simulink model "CORDIC_SAP"  (R2021a)
settings: Solver=VariableStepAuto  StartTime=0.0  StopTime=10.0  RelTol=1e-3
undefined symbols (not defined in the file or in its folder): AXI4, Lite
libraries: hdlBasic x278, xbsIndex_r4 x1
(part 3 of 3)

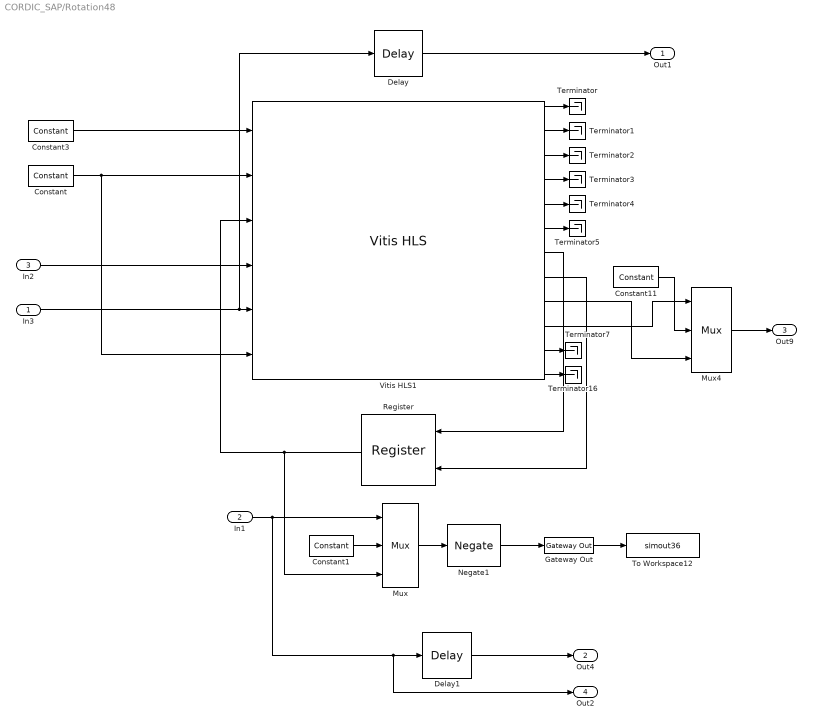
== system CORDIC_SAP/Rotation48 ==
  In3 : Inport
  In1 : Inport  Port=2
  In2 : Inport  Port=3
  Constant : hdlBasic/Constant  const=1.0  gui_display_data_type=Boolean  arith_type=Boolean  n_bits=16  bin_pt=14  preci_type=Single  exp_width=8  frac_width=24  explicit_period=off  period=1  XmcBlockStatus=1  maskContainerNames=tabcontainer1  block_type=constant  block_config=sysgen:Constant_config
  Constant1 : hdlBasic/Constant  const=0  gui_display_data_type=Fixed-point  arith_type=Signed (2's comp)  n_bits=16  bin_pt=13  preci_type=Single  exp_width=8  frac_width=24  explicit_period=off  period=1  XmcBlockStatus=1  maskContainerNames=tabcontainer1  block_type=constant  block_config=sysgen:Constant_config
  Constant11 : hdlBasic/Constant  const=0  gui_display_data_type=Fixed-point  arith_type=Signed (2's comp)  n_bits=16  bin_pt=13  preci_type=Single  exp_width=8  frac_width=24  explicit_period=off  period=1  XmcBlockStatus=1  maskContainerNames=tabcontainer1  block_type=constant  block_config=sysgen:Constant_config
  Constant3 : hdlBasic/Constant  const=0  gui_display_data_type=Boolean  arith_type=Boolean  n_bits=16  bin_pt=14  preci_type=Single  exp_width=8  frac_width=24  explicit_period=off  period=1  XmcBlockStatus=1  maskContainerNames=tabcontainer1  block_type=constant  block_config=sysgen:Constant_config
  Delay : hdlBasic/Delay  rst=off  en=off  latency=27  reg_retiming=off  XmcBlockStatus=1  maskContainerNames=group1  block_type=delay  block_config=sysgen:Delay_config
  Delay1 : hdlBasic/Delay  rst=off  en=off  latency=27  reg_retiming=off  XmcBlockStatus=1  maskContainerNames=group1  block_type=delay  block_config=sysgen:Delay_config
  Gateway Out : hdlBasic/Gateway Out  inherit_from_input=off  hdl_port=on  rows=1  columns=1  UseAsDAC=off  DACChannel='1'  interface=AXI4-Lite  automatic_assignment=on  address_offset=hex2dec('00')  intf_name=''  intf_description='Q_3_1'  timing_constraint=None  locs_specified=off  LOCs={}  io_standard={}  XmcBlockStatus=1  maskContainerNames=group4  block_type=gatewayout  block_config=sysgen:gateway_out_config  block_width_w=590  block_height_w=620  block_width=620  block_height=750
  Mux : hdlBasic/Mux  inputs=2  en=off  latency=1  precision=Full  arith_type=Unsigned  n_bits=16  bin_pt=14  quantization=Truncate  overflow=Wrap  XmcBlockStatus=1  maskContainerNames=tabcontainer1  block_type=mux  block_config=sysgen:Mux_config
  Mux4 : hdlBasic/Mux  inputs=2  en=off  latency=1  precision=Full  arith_type=Unsigned  n_bits=16  bin_pt=14  quantization=Truncate  overflow=Wrap  XmcBlockStatus=1  maskContainerNames=tabcontainer1  block_type=mux  block_config=sysgen:Mux_config
  Negate1 : hdlBasic/Negate  precision=Full  arith_type=Unsigned  n_bits=16  bin_pt=14  quantization=Truncate  overflow=Wrap  en=off  latency=0  XmcBlockStatus=1  maskContainerNames=tabcontainer1  block_type=negate  block_config=sysgen:Negate_config
  Register : hdlBasic/Register  init=0  rst=off  en=on  XmcBlockStatus=1  maskContainerNames=tabcontainer1  block_type=register  block_config=sysgen:Register_config
  Terminator{,1..5,7,16} (8 alike) : Terminator
  To Workspace12 : ToWorkspace  VariableName=simout36  SaveFormat=Timeseries  SampleTime=-1
  Vitis HLS1 : hdlBasic/Vitis HLS  anytable='C:\ELEC522\jz118\HLS\cordic\solution1'  fast_sim=off  display_datatype=off  rate_propagation_method=Simulink system period  model_file_path=''  latency=1  block_type=vitis_hls
      settings: infoedit=This block allows including C,C++ and SystemC source files in System Generator for DSP designs.
  Out1 : Outport
  Out4 : Outport  Port=2
  Out9 : Outport  Port=3
  Out2 : Outport  Port=4
  wires:
  In2/1 -> Vitis HLS1/4
  In3/1 -> Delay/1, Vitis HLS1/5
  Delay/1 -> Out1/1
  Constant/1 -> Vitis HLS1/2, Vitis HLS1/6
  Constant3/1 -> Vitis HLS1/1
  Vitis HLS1/1 -> Terminator/1
  Vitis HLS1/2 -> Terminator1/1
  Vitis HLS1/3 -> Terminator2/1
  Vitis HLS1/4 -> Terminator3/1
  Vitis HLS1/5 -> Terminator4/1
  Vitis HLS1/6 -> Terminator5/1
  Vitis HLS1/11 -> Terminator7/1
  Vitis HLS1/12 -> Terminator16/1
  Register/1 -> Mux/3, Vitis HLS1/3
  Vitis HLS1/8 -> Register/2
  Vitis HLS1/7 -> Register/1
  Constant11/1 -> Mux4/2
  Mux4/1 -> Out9/1
  Vitis HLS1/9 -> Mux4/3
  Vitis HLS1/10 -> Mux4/1
  In1/1 -> Out2/1, Delay1/1, Mux/1
  Constant1/1 -> Mux/2
  Mux/1 -> Negate1/1
  Negate1/1 -> Gateway Out/1
  Gateway Out/1 -> To Workspace12/1
  Delay1/1 -> Out4/1

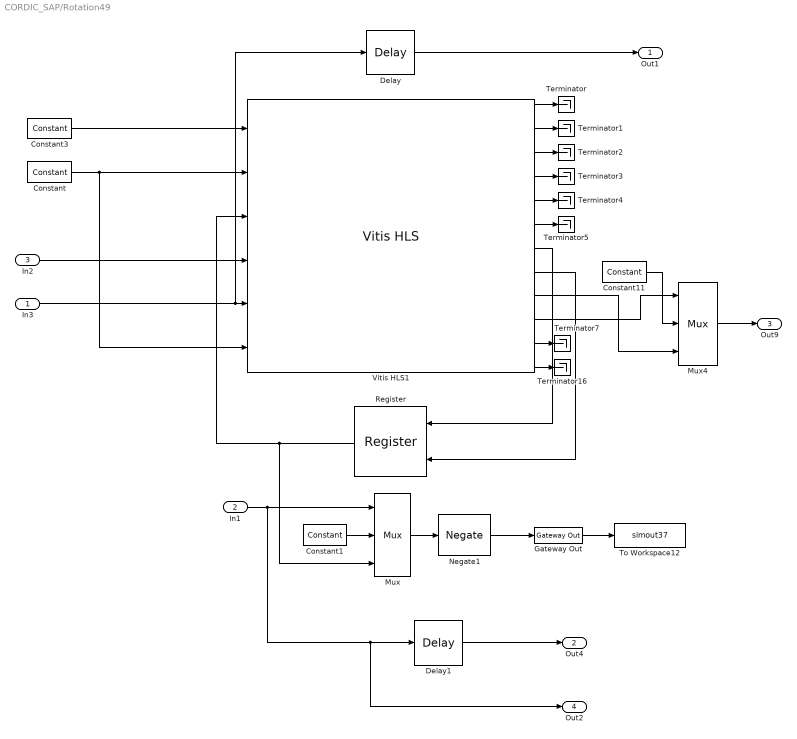
== system CORDIC_SAP/Rotation49 ==
  In3 : Inport
  In1 : Inport  Port=2
  In2 : Inport  Port=3
  Constant : hdlBasic/Constant  const=1.0  gui_display_data_type=Boolean  arith_type=Boolean  n_bits=16  bin_pt=14  preci_type=Single  exp_width=8  frac_width=24  explicit_period=off  period=1  XmcBlockStatus=1  maskContainerNames=tabcontainer1  block_type=constant  block_config=sysgen:Constant_config
  Constant1 : hdlBasic/Constant  const=0  gui_display_data_type=Fixed-point  arith_type=Signed (2's comp)  n_bits=16  bin_pt=13  preci_type=Single  exp_width=8  frac_width=24  explicit_period=off  period=1  XmcBlockStatus=1  maskContainerNames=tabcontainer1  block_type=constant  block_config=sysgen:Constant_config
  Constant11 : hdlBasic/Constant  const=0  gui_display_data_type=Fixed-point  arith_type=Signed (2's comp)  n_bits=16  bin_pt=13  preci_type=Single  exp_width=8  frac_width=24  explicit_period=off  period=1  XmcBlockStatus=1  maskContainerNames=tabcontainer1  block_type=constant  block_config=sysgen:Constant_config
  Constant3 : hdlBasic/Constant  const=0  gui_display_data_type=Boolean  arith_type=Boolean  n_bits=16  bin_pt=14  preci_type=Single  exp_width=8  frac_width=24  explicit_period=off  period=1  XmcBlockStatus=1  maskContainerNames=tabcontainer1  block_type=constant  block_config=sysgen:Constant_config
  Delay : hdlBasic/Delay  rst=off  en=off  latency=27  reg_retiming=off  XmcBlockStatus=1  maskContainerNames=group1  block_type=delay  block_config=sysgen:Delay_config
  Delay1 : hdlBasic/Delay  rst=off  en=off  latency=27  reg_retiming=off  XmcBlockStatus=1  maskContainerNames=group1  block_type=delay  block_config=sysgen:Delay_config
  Gateway Out : hdlBasic/Gateway Out  inherit_from_input=off  hdl_port=on  rows=1  columns=1  UseAsDAC=off  DACChannel='1'  interface=AXI4-Lite  automatic_assignment=on  address_offset=hex2dec('00')  intf_name=''  intf_description='Q_3_2'  timing_constraint=None  locs_specified=off  LOCs={}  io_standard={}  XmcBlockStatus=1  maskContainerNames=group4  block_type=gatewayout  block_config=sysgen:gateway_out_config  block_width_w=590  block_height_w=620  block_width=620  block_height=750
  Mux : hdlBasic/Mux  inputs=2  en=off  latency=1  precision=Full  arith_type=Unsigned  n_bits=16  bin_pt=14  quantization=Truncate  overflow=Wrap  XmcBlockStatus=1  maskContainerNames=tabcontainer1  block_type=mux  block_config=sysgen:Mux_config
  Mux4 : hdlBasic/Mux  inputs=2  en=off  latency=1  precision=Full  arith_type=Unsigned  n_bits=16  bin_pt=14  quantization=Truncate  overflow=Wrap  XmcBlockStatus=1  maskContainerNames=tabcontainer1  block_type=mux  block_config=sysgen:Mux_config
  Negate1 : hdlBasic/Negate  precision=Full  arith_type=Unsigned  n_bits=16  bin_pt=14  quantization=Truncate  overflow=Wrap  en=off  latency=0  XmcBlockStatus=1  maskContainerNames=tabcontainer1  block_type=negate  block_config=sysgen:Negate_config
  Register : hdlBasic/Register  init=0  rst=off  en=on  XmcBlockStatus=1  maskContainerNames=tabcontainer1  block_type=register  block_config=sysgen:Register_config
  Terminator{,1..5,7,16} (8 alike) : Terminator
  To Workspace12 : ToWorkspace  VariableName=simout37  SaveFormat=Timeseries  SampleTime=-1
  Vitis HLS1 : hdlBasic/Vitis HLS  anytable='C:\ELEC522\jz118\HLS\cordic\solution1'  fast_sim=off  display_datatype=off  rate_propagation_method=Simulink system period  model_file_path=''  latency=1  block_type=vitis_hls
      settings: infoedit=This block allows including C,C++ and SystemC source files in System Generator for DSP designs.
  Out1 : Outport
  Out4 : Outport  Port=2
  Out9 : Outport  Port=3
  Out2 : Outport  Port=4
  wires:
  In2/1 -> Vitis HLS1/4
  In3/1 -> Delay/1, Vitis HLS1/5
  Delay/1 -> Out1/1
  Constant/1 -> Vitis HLS1/2, Vitis HLS1/6
  Constant3/1 -> Vitis HLS1/1
  Vitis HLS1/1 -> Terminator/1
  Vitis HLS1/2 -> Terminator1/1
  Vitis HLS1/3 -> Terminator2/1
  Vitis HLS1/4 -> Terminator3/1
  Vitis HLS1/5 -> Terminator4/1
  Vitis HLS1/6 -> Terminator5/1
  Vitis HLS1/11 -> Terminator7/1
  Vitis HLS1/12 -> Terminator16/1
  Register/1 -> Mux/3, Vitis HLS1/3
  Vitis HLS1/8 -> Register/2
  Vitis HLS1/7 -> Register/1
  Constant11/1 -> Mux4/2
  Mux4/1 -> Out9/1
  Vitis HLS1/9 -> Mux4/3
  Vitis HLS1/10 -> Mux4/1
  In1/1 -> Out2/1, Delay1/1, Mux/1
  Constant1/1 -> Mux/2
  Mux/1 -> Negate1/1
  Negate1/1 -> Gateway Out/1
  Gateway Out/1 -> To Workspace12/1
  Delay1/1 -> Out4/1

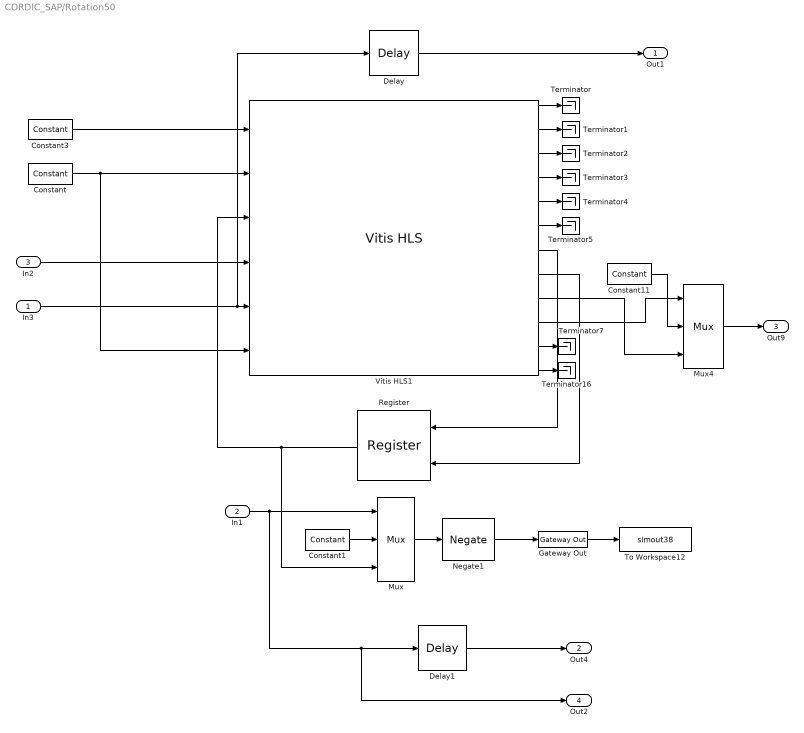
== system CORDIC_SAP/Rotation50 ==
  In3 : Inport
  In1 : Inport  Port=2
  In2 : Inport  Port=3
  Constant : hdlBasic/Constant  const=1.0  gui_display_data_type=Boolean  arith_type=Boolean  n_bits=16  bin_pt=14  preci_type=Single  exp_width=8  frac_width=24  explicit_period=off  period=1  XmcBlockStatus=1  maskContainerNames=tabcontainer1  block_type=constant  block_config=sysgen:Constant_config
  Constant1 : hdlBasic/Constant  const=0  gui_display_data_type=Fixed-point  arith_type=Signed (2's comp)  n_bits=16  bin_pt=13  preci_type=Single  exp_width=8  frac_width=24  explicit_period=off  period=1  XmcBlockStatus=1  maskContainerNames=tabcontainer1  block_type=constant  block_config=sysgen:Constant_config
  Constant11 : hdlBasic/Constant  const=0  gui_display_data_type=Fixed-point  arith_type=Signed (2's comp)  n_bits=16  bin_pt=13  preci_type=Single  exp_width=8  frac_width=24  explicit_period=off  period=1  XmcBlockStatus=1  maskContainerNames=tabcontainer1  block_type=constant  block_config=sysgen:Constant_config
  Constant3 : hdlBasic/Constant  const=0  gui_display_data_type=Boolean  arith_type=Boolean  n_bits=16  bin_pt=14  preci_type=Single  exp_width=8  frac_width=24  explicit_period=off  period=1  XmcBlockStatus=1  maskContainerNames=tabcontainer1  block_type=constant  block_config=sysgen:Constant_config
  Delay : hdlBasic/Delay  rst=off  en=off  latency=27  reg_retiming=off  XmcBlockStatus=1  maskContainerNames=group1  block_type=delay  block_config=sysgen:Delay_config
  Delay1 : hdlBasic/Delay  rst=off  en=off  latency=27  reg_retiming=off  XmcBlockStatus=1  maskContainerNames=group1  block_type=delay  block_config=sysgen:Delay_config
  Gateway Out : hdlBasic/Gateway Out  inherit_from_input=off  hdl_port=on  rows=1  columns=1  UseAsDAC=off  DACChannel='1'  interface=AXI4-Lite  automatic_assignment=on  address_offset=hex2dec('00')  intf_name=''  intf_description='Q_3_3'  timing_constraint=None  locs_specified=off  LOCs={}  io_standard={}  XmcBlockStatus=1  maskContainerNames=group4  block_type=gatewayout  block_config=sysgen:gateway_out_config  block_width_w=590  block_height_w=620  block_width=620  block_height=750
  Mux : hdlBasic/Mux  inputs=2  en=off  latency=1  precision=Full  arith_type=Unsigned  n_bits=16  bin_pt=14  quantization=Truncate  overflow=Wrap  XmcBlockStatus=1  maskContainerNames=tabcontainer1  block_type=mux  block_config=sysgen:Mux_config
  Mux4 : hdlBasic/Mux  inputs=2  en=off  latency=1  precision=Full  arith_type=Unsigned  n_bits=16  bin_pt=14  quantization=Truncate  overflow=Wrap  XmcBlockStatus=1  maskContainerNames=tabcontainer1  block_type=mux  block_config=sysgen:Mux_config
  Negate1 : hdlBasic/Negate  precision=Full  arith_type=Unsigned  n_bits=16  bin_pt=14  quantization=Truncate  overflow=Wrap  en=off  latency=0  XmcBlockStatus=1  maskContainerNames=tabcontainer1  block_type=negate  block_config=sysgen:Negate_config
  Register : hdlBasic/Register  init=0  rst=off  en=on  XmcBlockStatus=1  maskContainerNames=tabcontainer1  block_type=register  block_config=sysgen:Register_config
  Terminator{,1..5,7,16} (8 alike) : Terminator
  To Workspace12 : ToWorkspace  VariableName=simout38  SaveFormat=Timeseries  SampleTime=-1
  Vitis HLS1 : hdlBasic/Vitis HLS  anytable='C:\ELEC522\jz118\HLS\cordic\solution1'  fast_sim=off  display_datatype=off  rate_propagation_method=Simulink system period  model_file_path=''  latency=1  block_type=vitis_hls
      settings: infoedit=This block allows including C,C++ and SystemC source files in System Generator for DSP designs.
  Out1 : Outport
  Out4 : Outport  Port=2
  Out9 : Outport  Port=3
  Out2 : Outport  Port=4
  wires:
  In2/1 -> Vitis HLS1/4
  In3/1 -> Delay/1, Vitis HLS1/5
  Delay/1 -> Out1/1
  Constant/1 -> Vitis HLS1/2, Vitis HLS1/6
  Constant3/1 -> Vitis HLS1/1
  Vitis HLS1/1 -> Terminator/1
  Vitis HLS1/2 -> Terminator1/1
  Vitis HLS1/3 -> Terminator2/1
  Vitis HLS1/4 -> Terminator3/1
  Vitis HLS1/5 -> Terminator4/1
  Vitis HLS1/6 -> Terminator5/1
  Vitis HLS1/11 -> Terminator7/1
  Vitis HLS1/12 -> Terminator16/1
  Register/1 -> Mux/3, Vitis HLS1/3
  Vitis HLS1/8 -> Register/2
  Vitis HLS1/7 -> Register/1
  Constant11/1 -> Mux4/2
  Mux4/1 -> Out9/1
  Vitis HLS1/9 -> Mux4/3
  Vitis HLS1/10 -> Mux4/1
  In1/1 -> Out2/1, Delay1/1, Mux/1
  Constant1/1 -> Mux/2
  Mux/1 -> Negate1/1
  Negate1/1 -> Gateway Out/1
  Gateway Out/1 -> To Workspace12/1
  Delay1/1 -> Out4/1

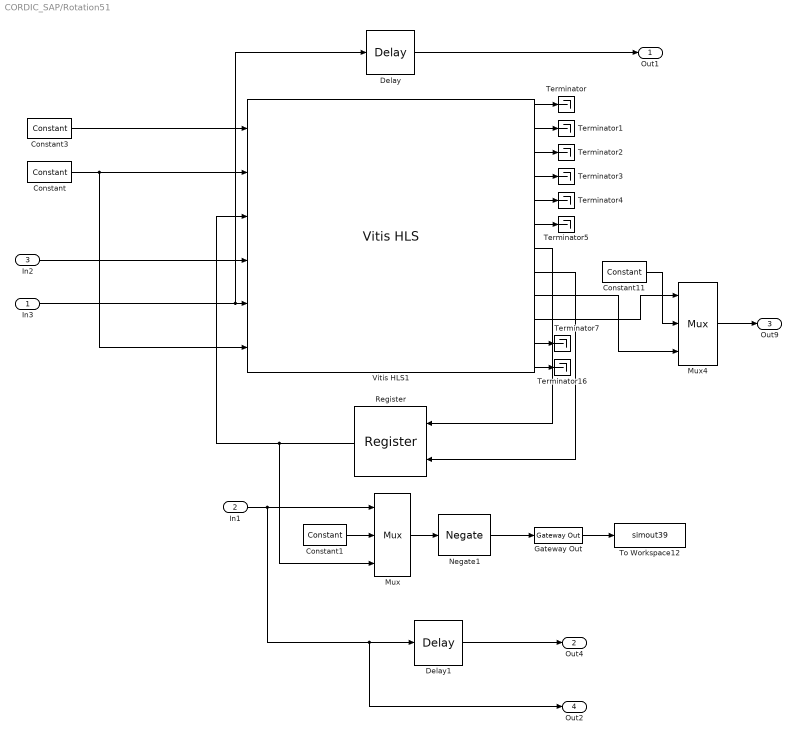
== system CORDIC_SAP/Rotation51 ==
  In3 : Inport
  In1 : Inport  Port=2
  In2 : Inport  Port=3
  Constant : hdlBasic/Constant  const=1.0  gui_display_data_type=Boolean  arith_type=Boolean  n_bits=16  bin_pt=14  preci_type=Single  exp_width=8  frac_width=24  explicit_period=off  period=1  XmcBlockStatus=1  maskContainerNames=tabcontainer1  block_type=constant  block_config=sysgen:Constant_config
  Constant1 : hdlBasic/Constant  const=0  gui_display_data_type=Fixed-point  arith_type=Signed (2's comp)  n_bits=16  bin_pt=13  preci_type=Single  exp_width=8  frac_width=24  explicit_period=off  period=1  XmcBlockStatus=1  maskContainerNames=tabcontainer1  block_type=constant  block_config=sysgen:Constant_config
  Constant11 : hdlBasic/Constant  const=0  gui_display_data_type=Fixed-point  arith_type=Signed (2's comp)  n_bits=16  bin_pt=13  preci_type=Single  exp_width=8  frac_width=24  explicit_period=off  period=1  XmcBlockStatus=1  maskContainerNames=tabcontainer1  block_type=constant  block_config=sysgen:Constant_config
  Constant3 : hdlBasic/Constant  const=0  gui_display_data_type=Boolean  arith_type=Boolean  n_bits=16  bin_pt=14  preci_type=Single  exp_width=8  frac_width=24  explicit_period=off  period=1  XmcBlockStatus=1  maskContainerNames=tabcontainer1  block_type=constant  block_config=sysgen:Constant_config
  Delay : hdlBasic/Delay  rst=off  en=off  latency=27  reg_retiming=off  XmcBlockStatus=1  maskContainerNames=group1  block_type=delay  block_config=sysgen:Delay_config
  Delay1 : hdlBasic/Delay  rst=off  en=off  latency=27  reg_retiming=off  XmcBlockStatus=1  maskContainerNames=group1  block_type=delay  block_config=sysgen:Delay_config
  Gateway Out : hdlBasic/Gateway Out  inherit_from_input=off  hdl_port=on  rows=1  columns=1  UseAsDAC=off  DACChannel='1'  interface=AXI4-Lite  automatic_assignment=on  address_offset=hex2dec('00')  intf_name=''  intf_description='Q_3_4'  timing_constraint=None  locs_specified=off  LOCs={}  io_standard={}  XmcBlockStatus=1  maskContainerNames=group4  block_type=gatewayout  block_config=sysgen:gateway_out_config  block_width_w=590  block_height_w=620  block_width=620  block_height=750
  Mux : hdlBasic/Mux  inputs=2  en=off  latency=1  precision=Full  arith_type=Unsigned  n_bits=16  bin_pt=14  quantization=Truncate  overflow=Wrap  XmcBlockStatus=1  maskContainerNames=tabcontainer1  block_type=mux  block_config=sysgen:Mux_config
  Mux4 : hdlBasic/Mux  inputs=2  en=off  latency=1  precision=Full  arith_type=Unsigned  n_bits=16  bin_pt=14  quantization=Truncate  overflow=Wrap  XmcBlockStatus=1  maskContainerNames=tabcontainer1  block_type=mux  block_config=sysgen:Mux_config
  Negate1 : hdlBasic/Negate  precision=Full  arith_type=Unsigned  n_bits=16  bin_pt=14  quantization=Truncate  overflow=Wrap  en=off  latency=0  XmcBlockStatus=1  maskContainerNames=tabcontainer1  block_type=negate  block_config=sysgen:Negate_config
  Register : hdlBasic/Register  init=0  rst=off  en=on  XmcBlockStatus=1  maskContainerNames=tabcontainer1  block_type=register  block_config=sysgen:Register_config
  Terminator{,1..5,7,16} (8 alike) : Terminator
  To Workspace12 : ToWorkspace  VariableName=simout39  SaveFormat=Timeseries  SampleTime=-1
  Vitis HLS1 : hdlBasic/Vitis HLS  anytable='C:\ELEC522\jz118\HLS\cordic\solution1'  fast_sim=off  display_datatype=off  rate_propagation_method=Simulink system period  model_file_path=''  latency=1  block_type=vitis_hls
      settings: infoedit=This block allows including C,C++ and SystemC source files in System Generator for DSP designs.
  Out1 : Outport
  Out4 : Outport  Port=2
  Out9 : Outport  Port=3
  Out2 : Outport  Port=4
  wires:
  In2/1 -> Vitis HLS1/4
  In3/1 -> Delay/1, Vitis HLS1/5
  Delay/1 -> Out1/1
  Constant/1 -> Vitis HLS1/2, Vitis HLS1/6
  Constant3/1 -> Vitis HLS1/1
  Vitis HLS1/1 -> Terminator/1
  Vitis HLS1/2 -> Terminator1/1
  Vitis HLS1/3 -> Terminator2/1
  Vitis HLS1/4 -> Terminator3/1
  Vitis HLS1/5 -> Terminator4/1
  Vitis HLS1/6 -> Terminator5/1
  Vitis HLS1/11 -> Terminator7/1
  Vitis HLS1/12 -> Terminator16/1
  Register/1 -> Mux/3, Vitis HLS1/3
  Vitis HLS1/8 -> Register/2
  Vitis HLS1/7 -> Register/1
  Constant11/1 -> Mux4/2
  Mux4/1 -> Out9/1
  Vitis HLS1/9 -> Mux4/3
  Vitis HLS1/10 -> Mux4/1
  In1/1 -> Out2/1, Delay1/1, Mux/1
  Constant1/1 -> Mux/2
  Mux/1 -> Negate1/1
  Negate1/1 -> Gateway Out/1
  Gateway Out/1 -> To Workspace12/1
  Delay1/1 -> Out4/1

== system CORDIC_SAP/Vectoring12 ==
  In1 : Inport
  In2 : Inport  Port=2
  Constant1 : hdlBasic/Constant  const=0  gui_display_data_type=Fixed-point  arith_type=Signed (2's comp)  n_bits=16  bin_pt=13  preci_type=Single  exp_width=8  frac_width=24  explicit_period=off  period=1  XmcBlockStatus=1  maskContainerNames=tabcontainer1  block_type=constant  block_config=sysgen:Constant_config
  Constant10 : hdlBasic/Constant  const=0  gui_display_data_type=Fixed-point  arith_type=Signed (2's comp)  n_bits=16  bin_pt=13  preci_type=Single  exp_width=8  frac_width=24  explicit_period=off  period=1  XmcBlockStatus=1  maskContainerNames=tabcontainer1  block_type=constant  block_config=sysgen:Constant_config
  Constant11 : hdlBasic/Constant  const=0  gui_display_data_type=Fixed-point  arith_type=Signed (2's comp)  n_bits=16  bin_pt=13  preci_type=Single  exp_width=8  frac_width=24  explicit_period=off  period=1  XmcBlockStatus=1  maskContainerNames=tabcontainer1  block_type=constant  block_config=sysgen:Constant_config
  Constant8 : hdlBasic/Constant  const=0  gui_display_data_type=Boolean  arith_type=Boolean  n_bits=16  bin_pt=13  preci_type=Single  exp_width=8  frac_width=24  explicit_period=off  period=1  XmcBlockStatus=1  maskContainerNames=tabcontainer1  block_type=constant  block_config=sysgen:Constant_config
  Constant9 : hdlBasic/Constant  const=1  gui_display_data_type=Boolean  arith_type=Boolean  n_bits=16  bin_pt=13  preci_type=Single  exp_width=8  frac_width=24  explicit_period=off  period=1  XmcBlockStatus=1  maskContainerNames=tabcontainer1  block_type=constant  block_config=sysgen:Constant_config
  Delay : hdlBasic/Delay  rst=off  en=off  latency=27  reg_retiming=off  XmcBlockStatus=1  maskContainerNames=group1  block_type=delay  block_config=sysgen:Delay_config
  Gateway Out43 : hdlBasic/Gateway Out  inherit_from_input=off  hdl_port=on  rows=1  columns=1  UseAsDAC=off  DACChannel='1'  interface=AXI4-Lite  automatic_assignment=on  address_offset=hex2dec('00')  intf_name=''  intf_description='R_3_3'  timing_constraint=None  locs_specified=off  LOCs={}  io_standard={}  XmcBlockStatus=1  maskContainerNames=group4  block_type=gatewayout  block_config=sysgen:gateway_out_config  block_width_w=590  block_height_w=620  block_width=620  block_height=750
  Mux : hdlBasic/Mux  inputs=2  en=off  latency=1  precision=Full  arith_type=Unsigned  n_bits=16  bin_pt=14  quantization=Truncate  overflow=Wrap  XmcBlockStatus=1  maskContainerNames=tabcontainer1  block_type=mux  block_config=sysgen:Mux_config
  Mux4 : hdlBasic/Mux  inputs=2  en=off  latency=1  precision=Full  arith_type=Unsigned  n_bits=16  bin_pt=14  quantization=Truncate  overflow=Wrap  XmcBlockStatus=1  maskContainerNames=tabcontainer1  block_type=mux  block_config=sysgen:Mux_config
  Register : hdlBasic/Register  init=0  rst=off  en=on  XmcBlockStatus=1  maskContainerNames=tabcontainer1  block_type=register  block_config=sysgen:Register_config
  Scope : Scope  NumInputPorts=2
  Terminator{8..15} (8 alike) : Terminator
  To Workspace12 : ToWorkspace  VariableName=simout26  SaveFormat=Timeseries  SampleTime=-1
  Vitis HLS2 : hdlBasic/Vitis HLS  anytable='C:\ELEC522\jz118\HLS\cordic\solution1'  fast_sim=off  display_datatype=off  rate_propagation_method=Simulink system period  model_file_path=''  latency=1  block_type=vitis_hls
      settings: infoedit=This block allows including C,C++ and SystemC source files in System Generator for DSP designs.
  Out1 : Outport
  Out3 : Outport  Port=2
  wires:
  Vitis HLS2/9 -> Terminator14/1
  Vitis HLS2/5 -> Terminator9/1
  Vitis HLS2/2 -> Terminator10/1
  Vitis HLS2/4 -> Terminator12/1
  Vitis HLS2/6 -> Terminator8/1
  Vitis HLS2/10 -> Terminator15/1
  Constant8/1 -> Vitis HLS2/1, Vitis HLS2/6
  Constant9/1 -> Vitis HLS2/2
  Vitis HLS2/3 -> Terminator11/1
  Vitis HLS2/1 -> Terminator13/1
  Constant10/1 -> Vitis HLS2/5
  In2/1 -> Scope/1, Vitis HLS2/4
  Vitis HLS2/7 -> Register/1
  Vitis HLS2/8 -> Register/2
  Register/1 -> Mux/3, Scope/2, Vitis HLS2/3
  Constant11/1 -> Mux4/2
  Mux4/1 -> Out1/1
  Vitis HLS2/12 -> Mux4/1
  Vitis HLS2/11 -> Mux4/3
  In1/1 -> Delay/1, Mux/1
  Constant1/1 -> Mux/2
  Delay/1 -> Out3/1
  Mux/1 -> Gateway Out43/1
  Gateway Out43/1 -> To Workspace12/1

== system CORDIC_SAP/Vectoring14 ==
  In1 : Inport
  In2 : Inport  Port=2
  Constant1 : hdlBasic/Constant  const=0  gui_display_data_type=Fixed-point  arith_type=Signed (2's comp)  n_bits=16  bin_pt=13  preci_type=Single  exp_width=8  frac_width=24  explicit_period=off  period=1  XmcBlockStatus=1  maskContainerNames=tabcontainer1  block_type=constant  block_config=sysgen:Constant_config
  Constant10 : hdlBasic/Constant  const=0  gui_display_data_type=Fixed-point  arith_type=Signed (2's comp)  n_bits=16  bin_pt=13  preci_type=Single  exp_width=8  frac_width=24  explicit_period=off  period=1  XmcBlockStatus=1  maskContainerNames=tabcontainer1  block_type=constant  block_config=sysgen:Constant_config
  Constant11 : hdlBasic/Constant  const=0  gui_display_data_type=Fixed-point  arith_type=Signed (2's comp)  n_bits=16  bin_pt=13  preci_type=Single  exp_width=8  frac_width=24  explicit_period=off  period=1  XmcBlockStatus=1  maskContainerNames=tabcontainer1  block_type=constant  block_config=sysgen:Constant_config
  Constant8 : hdlBasic/Constant  const=0  gui_display_data_type=Boolean  arith_type=Boolean  n_bits=16  bin_pt=13  preci_type=Single  exp_width=8  frac_width=24  explicit_period=off  period=1  XmcBlockStatus=1  maskContainerNames=tabcontainer1  block_type=constant  block_config=sysgen:Constant_config
  Constant9 : hdlBasic/Constant  const=1  gui_display_data_type=Boolean  arith_type=Boolean  n_bits=16  bin_pt=13  preci_type=Single  exp_width=8  frac_width=24  explicit_period=off  period=1  XmcBlockStatus=1  maskContainerNames=tabcontainer1  block_type=constant  block_config=sysgen:Constant_config
  Delay : hdlBasic/Delay  rst=off  en=off  latency=27  reg_retiming=off  XmcBlockStatus=1  maskContainerNames=group1  block_type=delay  block_config=sysgen:Delay_config
  Gateway Out43 : hdlBasic/Gateway Out  inherit_from_input=off  hdl_port=on  rows=1  columns=1  UseAsDAC=off  DACChannel='1'  interface=AXI4-Lite  automatic_assignment=on  address_offset=hex2dec('00')  intf_name=''  intf_description='R1_1'  timing_constraint=None  locs_specified=off  LOCs={}  io_standard={}  XmcBlockStatus=1  maskContainerNames=group4  block_type=gatewayout  block_config=sysgen:gateway_out_config  block_width_w=590  block_height_w=620  block_width=620  block_height=750
  Mux : hdlBasic/Mux  inputs=2  en=off  latency=1  precision=Full  arith_type=Unsigned  n_bits=16  bin_pt=14  quantization=Truncate  overflow=Wrap  XmcBlockStatus=1  maskContainerNames=tabcontainer1  block_type=mux  block_config=sysgen:Mux_config
  Mux4 : hdlBasic/Mux  inputs=2  en=off  latency=1  precision=Full  arith_type=Unsigned  n_bits=16  bin_pt=14  quantization=Truncate  overflow=Wrap  XmcBlockStatus=1  maskContainerNames=tabcontainer1  block_type=mux  block_config=sysgen:Mux_config
  Register : hdlBasic/Register  init=0  rst=off  en=on  XmcBlockStatus=1  maskContainerNames=tabcontainer1  block_type=register  block_config=sysgen:Register_config
  Terminator{8..15} (8 alike) : Terminator
  To Workspace12 : ToWorkspace  VariableName=simout12  SaveFormat=Timeseries  SampleTime=-1
  Vitis HLS2 : hdlBasic/Vitis HLS  anytable='C:\ELEC522\jz118\HLS\cordic\solution1'  fast_sim=off  display_datatype=off  rate_propagation_method=Simulink system period  model_file_path=''  latency=1  block_type=vitis_hls
      settings: infoedit=This block allows including C,C++ and SystemC source files in System Generator for DSP designs.
  Out1 : Outport
  Out3 : Outport  Port=2
  wires:
  Vitis HLS2/9 -> Terminator14/1
  Vitis HLS2/5 -> Terminator9/1
  Vitis HLS2/2 -> Terminator10/1
  Vitis HLS2/4 -> Terminator12/1
  Vitis HLS2/6 -> Terminator8/1
  Vitis HLS2/10 -> Terminator15/1
  Constant8/1 -> Vitis HLS2/1, Vitis HLS2/6
  Constant9/1 -> Vitis HLS2/2
  Vitis HLS2/3 -> Terminator11/1
  Vitis HLS2/1 -> Terminator13/1
  Constant10/1 -> Vitis HLS2/5
  In2/1 -> Vitis HLS2/4
  Vitis HLS2/7 -> Register/1
  Vitis HLS2/8 -> Register/2
  Register/1 -> Mux/3, Vitis HLS2/3
  Constant11/1 -> Mux4/2
  Mux4/1 -> Out1/1
  Vitis HLS2/11 -> Mux4/3
  In1/1 -> Delay/1, Mux/1
  Constant1/1 -> Mux/2
  Delay/1 -> Out3/1
  Gateway Out43/1 -> To Workspace12/1
  Mux/1 -> Gateway Out43/1
  Vitis HLS2/12 -> Mux4/1

== system CORDIC_SAP/Vectoring15 ==
  In1 : Inport
  In2 : Inport  Port=2
  Constant1 : hdlBasic/Constant  const=0  gui_display_data_type=Fixed-point  arith_type=Signed (2's comp)  n_bits=16  bin_pt=13  preci_type=Single  exp_width=8  frac_width=24  explicit_period=off  period=1  XmcBlockStatus=1  maskContainerNames=tabcontainer1  block_type=constant  block_config=sysgen:Constant_config
  Constant10 : hdlBasic/Constant  const=0  gui_display_data_type=Fixed-point  arith_type=Signed (2's comp)  n_bits=16  bin_pt=13  preci_type=Single  exp_width=8  frac_width=24  explicit_period=off  period=1  XmcBlockStatus=1  maskContainerNames=tabcontainer1  block_type=constant  block_config=sysgen:Constant_config
  Constant11 : hdlBasic/Constant  const=0  gui_display_data_type=Fixed-point  arith_type=Signed (2's comp)  n_bits=16  bin_pt=13  preci_type=Single  exp_width=8  frac_width=24  explicit_period=off  period=1  XmcBlockStatus=1  maskContainerNames=tabcontainer1  block_type=constant  block_config=sysgen:Constant_config
  Constant8 : hdlBasic/Constant  const=0  gui_display_data_type=Boolean  arith_type=Boolean  n_bits=16  bin_pt=13  preci_type=Single  exp_width=8  frac_width=24  explicit_period=off  period=1  XmcBlockStatus=1  maskContainerNames=tabcontainer1  block_type=constant  block_config=sysgen:Constant_config
  Constant9 : hdlBasic/Constant  const=1  gui_display_data_type=Boolean  arith_type=Boolean  n_bits=16  bin_pt=13  preci_type=Single  exp_width=8  frac_width=24  explicit_period=off  period=1  XmcBlockStatus=1  maskContainerNames=tabcontainer1  block_type=constant  block_config=sysgen:Constant_config
  Delay : hdlBasic/Delay  rst=off  en=off  latency=27  reg_retiming=off  XmcBlockStatus=1  maskContainerNames=group1  block_type=delay  block_config=sysgen:Delay_config
  Gateway Out43 : hdlBasic/Gateway Out  inherit_from_input=off  hdl_port=on  rows=1  columns=1  UseAsDAC=off  DACChannel='1'  interface=AXI4-Lite  automatic_assignment=on  address_offset=hex2dec('00')  intf_name=''  intf_description='R_2_2'  timing_constraint=None  locs_specified=off  LOCs={}  io_standard={}  XmcBlockStatus=1  maskContainerNames=group4  block_type=gatewayout  block_config=sysgen:gateway_out_config  block_width_w=590  block_height_w=620  block_width=620  block_height=750
  Mux : hdlBasic/Mux  inputs=2  en=off  latency=1  precision=Full  arith_type=Unsigned  n_bits=16  bin_pt=14  quantization=Truncate  overflow=Wrap  XmcBlockStatus=1  maskContainerNames=tabcontainer1  block_type=mux  block_config=sysgen:Mux_config
  Mux4 : hdlBasic/Mux  inputs=2  en=off  latency=1  precision=Full  arith_type=Unsigned  n_bits=16  bin_pt=14  quantization=Truncate  overflow=Wrap  XmcBlockStatus=1  maskContainerNames=tabcontainer1  block_type=mux  block_config=sysgen:Mux_config
  Register : hdlBasic/Register  init=0  rst=off  en=on  XmcBlockStatus=1  maskContainerNames=tabcontainer1  block_type=register  block_config=sysgen:Register_config
  Terminator{8..15} (8 alike) : Terminator
  To Workspace12 : ToWorkspace  VariableName=simout23  SaveFormat=Timeseries  SampleTime=-1
  Vitis HLS2 : hdlBasic/Vitis HLS  anytable='C:\ELEC522\jz118\HLS\cordic\solution1'  fast_sim=off  display_datatype=off  rate_propagation_method=Simulink system period  model_file_path=''  latency=1  block_type=vitis_hls
      settings: infoedit=This block allows including C,C++ and SystemC source files in System Generator for DSP designs.
  Out1 : Outport
  Out3 : Outport  Port=2
  wires:
  Vitis HLS2/9 -> Terminator14/1
  Vitis HLS2/5 -> Terminator9/1
  Vitis HLS2/2 -> Terminator10/1
  Vitis HLS2/4 -> Terminator12/1
  Vitis HLS2/6 -> Terminator8/1
  Vitis HLS2/10 -> Terminator15/1
  Constant8/1 -> Vitis HLS2/1, Vitis HLS2/6
  Constant9/1 -> Vitis HLS2/2
  Vitis HLS2/3 -> Terminator11/1
  Vitis HLS2/1 -> Terminator13/1
  Constant10/1 -> Vitis HLS2/5
  In2/1 -> Vitis HLS2/4
  Vitis HLS2/7 -> Register/1
  Vitis HLS2/8 -> Register/2
  Register/1 -> Mux/3, Vitis HLS2/3
  Constant11/1 -> Mux4/2
  Mux4/1 -> Out1/1
  Vitis HLS2/11 -> Mux4/3
  In1/1 -> Delay/1, Mux/1
  Constant1/1 -> Mux/2
  Delay/1 -> Out3/1
  Gateway Out43/1 -> To Workspace12/1
  Mux/1 -> Gateway Out43/1
  Vitis HLS2/12 -> Mux4/1
